simulink model "testmodel"  (R2023b)
settings: Solver=VariableStepAuto  StartTime=0.0  StopTime=10.0  RelTol=1e-3
settings Model: Creator=taku0  LastModifiedBy=taku0

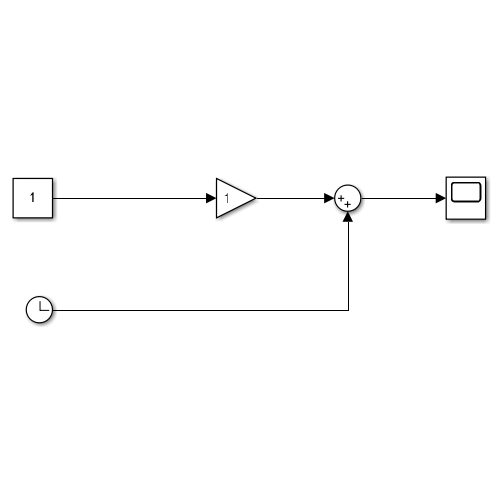
[thumbnail: Simulink's stored preview of the top-level diagram]
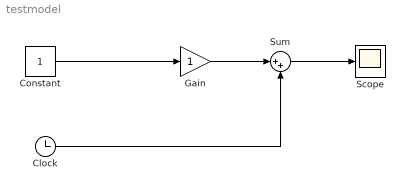
== system testmodel ==
  Clock : Clock
  Constant : Constant
  Gain : Gain
  Scope : Scope
  Sum : Sum  Inputs=|++
  wires:
  Constant/1 -> Gain/1
  Gain/1 -> Sum/1
  Clock/1 -> Sum/2
  Sum/1 -> Scope/1
